simulink model "model3_2"
settings: Solver=ode4  SolverMode=SingleTasking  StartTime=0.0  StopTime=10.0  FixedStep=0.01  RelTol=1e-3
values from neighbouring files (symbols this model uses):
  A = [0 1; -I -N]    [lab3_2.m]
  A_p = expm(h*A)    [lab3_2.m]
  B = [0; 1]    [lab3_2.m]
  B_p = double(int(expm(A*t)*B,t,0,h))    [lab3_2.m]
  C = eye(2)    [lab3_2.m]
  C_p = C    [lab3_2.m]
  D = [0; 0]    [lab3_2.m]
  D_p = D    [lab3_2.m]
  h = 0.1    [lab3_2.m]
  WPC = 2    [lab3_1.m]    (also in lab3_2.m = 1)
settings Model: Creator=Dell  LastModifiedBy=student
settings DataIOCC: LimitDataPoints=on  SaveFormat=Array  SignalLoggingSaveFormat=ModelDataLogs  ReturnWorkspaceOutputs=off
settings OptimizationCC: BlockReduction=off  BooleanDataType=off  ExpressionDepthLimit=2147483647  LifeSpan=inf  SimCompilerOptimization=Off
settings DebuggingCC: SaveWithParameterizedLinksMsg=none  UnderspecifiedInitializationDetection=Classic  MergeDetectMultiDrivingBlocksExec=none  SignalResolutionControl=TryResolveAllWithWarning  MultiTaskDSMMsg=warning  MultiTaskCondExecSysMsg=none  FcnCallInpInsideContextMsg=Enable All  FrameProcessingCompatibilityMsg=warning  StateNameClashWarn=warning  StrictBusMsg=None  SFUnexpectedBacktrackingDiag=warning  SFNoUnconditionalDefaultTransitionDiag=warning
settings HardwareCC: ProdBitPerPointer=32  ProdLargestAtomicFloat=None  ProdIntDivRoundTo=Undefined  ProdEndianess=Unspecified  ProdWordSize=32  ProdHWDeviceType=32-bit Generic  TargetUnknown=on
settings ModelReferenceCC: PropagateSignalLabelsOutOfModel=off
settings SFSimCC: SimUseLocalCustomCode=off
settings RTWCC: RTWUseLocalCustomCode=off  IncludeERTFirstTime=on  RTWCompilerOptimization=Off
settings CodeAppCC: CustomSymbolStrType=$N$R$M
settings GRTTargetCC: CodeReplacementLibrary=ANSI_C  GeneratePreprocessorConditionals=Disable all  CPPClassGenCompliant=off

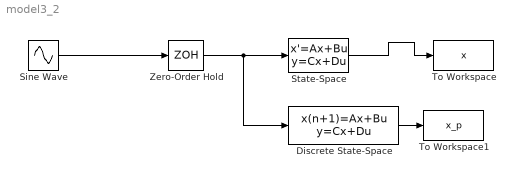
== system model3_2 ==
  Discrete State-Space : DiscreteStateSpace  A=A_p  B=B_p  C=C_p  D=D_p  X0=WPC  SampleTime=h
  Sine Wave : Sin  SampleTime=0
  State-Space : StateSpace  A=A  B=B  C=C  D=D  X0=WPC
  To Workspace : ToWorkspace  VariableName=x  SampleTime=h  SaveFormat=Timeseries
  To Workspace1 : ToWorkspace  VariableName=x_p  SampleTime=h  SaveFormat=Timeseries
  Zero-Order Hold : ZeroOrderHold  SampleTime=h
  wires:
  Sine Wave/1 -> Zero-Order Hold/1
  Zero-Order Hold/1 -> Discrete State-Space/1, State-Space/1
  State-Space/1 -> To Workspace/1
  Discrete State-Space/1 -> To Workspace1/1
